simulink model "WaveletTraj"  (Simulink 10.1)
settings: Solver=FixedStepDiscrete  StartTime=0.0  StopTime=inf  FixedStep=Ts  RelTol=1e-3
PreLoadFcn:
  | load param
undefined symbols (not defined in the file or in its folder): c_maxsz, DiscIntNeverNeededParam, Dphival_fi, f, interp_gain, interp_uplim, phival_fi, Ts, tval_fi, w
libraries: simulink x36, dspsigops x24, dspindex x16, dspswit3 x12, simulink_extras x8
(part 4 of 4)

== system WaveletTraj/Wavelet Trajectory/TrajGen4/Compute Outputs/Compute Integral ==
  x : Inport
  max : Inport  Port=2
  min : Inport  Port=3
  Enable : EnablePort
  Compare To Zero : simulink/Logic and Bit Operations/Compare To Zero  SystemSampleTime=-1  relop=<  LogicOutDataTypeMode=boolean  ZeroCross=off
  Compare To Zero1 : simulink/Logic and Bit Operations/Compare To Zero  SystemSampleTime=-1  relop=>  LogicOutDataTypeMode=boolean  ZeroCross=off
  Discrete-Time Integrator : DiscreteIntegrator  IntegratorMethod=Integration: Trapezoidal  ExternalReset=level  InitialConditionSource=external  SampleTime=Ts  OutDataTypeStr=fixdt(1,w,f)  RndMeth=Nearest  SaturateOnIntegerOverflow=on  ICPrevOutput=DiscIntNeverNeededParam  ICPrevScaledInput=DiscIntNeverNeededParam
  Logical Operator : Logic  Operator=OR  IconShape=distinctive  AllPortsSameDT=off  OutDataTypeStr=boolean
  Logical Operator1 : Logic  IconShape=distinctive  AllPortsSameDT=off  OutDataTypeStr=boolean
  Logical Operator2 : Logic  IconShape=distinctive  AllPortsSameDT=off  OutDataTypeStr=boolean
  Logical Operator3 : Logic  Operator=OR  IconShape=distinctive  AllPortsSameDT=off  OutDataTypeStr=boolean
  Relational Operator1 : RelationalOperator  Operator=<=  OutDataTypeStr=boolean  RndMeth=Nearest
  Relational Operator2 : RelationalOperator  Operator=<=  OutDataTypeStr=boolean  RndMeth=Nearest
  S-R Flip-Flop : simulink_extras/Flip Flops/S-R Flip-Flop  SystemSampleTime=-1  initial_condition=0
  Sample and Hold1 : dspsigops/Sample and Hold  SystemSampleTime=-1  trig=Either edge  initCond=0  latchinput=off
  Sample and Hold2 : dspsigops/Sample and Hold  SystemSampleTime=-1  trig=Either edge  initCond=0  latchinput=off
  Saturation Dynamic : simulink/Discontinuities/Saturation Dynamic  SystemSampleTime=-1  OutMin=[]  OutMax=[]  OutDataTypeStr=fixdt(1,w,f)  OutputDataTypeScalingMode=Specify via dialog  OutDataType=fixdt(1,w,f)  OutScaling=[]  RndMeth=Nearest  DoSatur=on
  Terminator : Terminator
  Unit Delay : UnitDelay  SampleTime=-1
  Ix : Outport
  wires:
  Sample and Hold2/1 -> Logical Operator2/1
  Sample and Hold1/1 -> Logical Operator1/1
  Logical Operator3/1 -> S-R Flip-Flop/2
  Logical Operator2/1 -> Logical Operator3/2
  Logical Operator1/1 -> Logical Operator3/1
  Compare To Zero1/1 -> Logical Operator2/2
  Compare To Zero/1 -> Logical Operator1/2
  Logical Operator/1 -> Sample and Hold2/Trigger, Sample and Hold1/Trigger, S-R Flip-Flop/1
  S-R Flip-Flop/2 -> Terminator/1
  S-R Flip-Flop/1 -> Discrete-Time Integrator/2
  Unit Delay/1 -> Relational Operator2/1, Relational Operator1/2, Discrete-Time Integrator/3
  x/1 -> Compare To Zero1/1, Compare To Zero/1, Discrete-Time Integrator/1
  Saturation Dynamic/1 -> Unit Delay/1, Ix/1
  Discrete-Time Integrator/1 -> Saturation Dynamic/2
  Relational Operator2/1 -> Logical Operator/2, Sample and Hold2/1
  Relational Operator1/1 -> Sample and Hold1/1, Logical Operator/1
  min/1 -> Saturation Dynamic/3, Relational Operator2/2
  max/1 -> Saturation Dynamic/1, Relational Operator1/1

== system WaveletTraj/Wavelet Trajectory/TrajGen4/Compute Outputs/Rate Limiter1 ==
  up : Inport
  u : Inport  Port=2
  lo : Inport  Port=3
  Gain : Gain  Gain=1/Ts  ParamDataTypeStr=fixdt(1,w,f)  RndMeth=Nearest  SaturateOnIntegerOverflow=on  OutDataTypeStr=Inherit: Same as input
  Gain1 : Gain  Gain=Ts  ParamDataTypeStr=fixdt(1,w,f)  OutDataTypeStr=fixdt(1,w,f)  RndMeth=Nearest  SaturateOnIntegerOverflow=on
  Gain2 : Gain  Gain=Ts  ParamDataTypeStr=fixdt(1,w,f)  OutDataTypeStr=fixdt(1,w,f)  RndMeth=Nearest  SaturateOnIntegerOverflow=on
  Relational Operator : RelationalOperator  Operator=<  OutDataTypeStr=boolean  RndMeth=Nearest
  Relational Operator1 : RelationalOperator  Operator=>  OutDataTypeStr=boolean  RndMeth=Nearest
  Sum1 : Sum  Inputs=|++  OutDataTypeStr=fixdt(1,w,f)  RndMeth=Nearest  SaturateOnIntegerOverflow=on
  Sum2 : Sum  Inputs=|+-  OutDataTypeStr=fixdt(1,w,f)  RndMeth=Nearest  SaturateOnIntegerOverflow=on
  Sum3 : Sum  Inputs=|++  OutDataTypeStr=fixdt(1,w,f)  RndMeth=Nearest  SaturateOnIntegerOverflow=on
  Switch1 : Switch  Threshold=0.5  OutDataTypeStr=fixdt(1,w,f)  RndMeth=Nearest  SaturateOnIntegerOverflow=on
  Switch2 : Switch  Threshold=0.5  OutDataTypeStr=fixdt(1,w,f)  RndMeth=Nearest  SaturateOnIntegerOverflow=on
  Unit Delay : UnitDelay  SampleTime=-1
  y : Outport
  wires:
  Sum3/1 -> Switch2/3
  Gain2/1 -> Sum3/1
  lo/1 -> Gain2/1, Relational Operator1/2
  Relational Operator1/1 -> Switch2/2
  Switch2/1 -> Unit Delay/1, y/1
  Switch1/1 -> Switch2/1
  Sum1/1 -> Switch1/1
  Gain1/1 -> Sum1/1
  Relational Operator/1 -> Switch1/2
  up/1 -> Gain1/1, Relational Operator/1
  Gain/1 -> Relational Operator1/1, Relational Operator/2
  Unit Delay/1 -> Sum3/2, Sum1/2, Sum2/2
  Sum2/1 -> Gain/1
  u/1 -> Switch1/3, Sum2/1

== system WaveletTraj/Wavelet Trajectory/TrajGen4/Compute Outputs/Rate Limiter2 ==
  up : Inport
  u : Inport  Port=2
  lo : Inport  Port=3
  Gain : Gain  Gain=1/Ts  ParamDataTypeStr=fixdt(1,w,f)  RndMeth=Nearest  SaturateOnIntegerOverflow=on  OutDataTypeStr=Inherit: Same as input
  Gain1 : Gain  Gain=Ts  ParamDataTypeStr=fixdt(1,w,f)  OutDataTypeStr=fixdt(1,w,f)  RndMeth=Nearest  SaturateOnIntegerOverflow=on
  Gain2 : Gain  Gain=Ts  ParamDataTypeStr=fixdt(1,w,f)  OutDataTypeStr=fixdt(1,w,f)  RndMeth=Nearest  SaturateOnIntegerOverflow=on
  Relational Operator : RelationalOperator  Operator=<  OutDataTypeStr=boolean  RndMeth=Nearest
  Relational Operator1 : RelationalOperator  Operator=>  OutDataTypeStr=boolean  RndMeth=Nearest
  Sum1 : Sum  Inputs=|++  OutDataTypeStr=fixdt(1,w,f)  RndMeth=Nearest  SaturateOnIntegerOverflow=on
  Sum2 : Sum  Inputs=|+-  OutDataTypeStr=fixdt(1,w,f)  RndMeth=Nearest  SaturateOnIntegerOverflow=on
  Sum3 : Sum  Inputs=|++  OutDataTypeStr=fixdt(1,w,f)  RndMeth=Nearest  SaturateOnIntegerOverflow=on
  Switch1 : Switch  Threshold=0.5  OutDataTypeStr=fixdt(1,w,f)  RndMeth=Nearest  SaturateOnIntegerOverflow=on
  Switch2 : Switch  Threshold=0.5  OutDataTypeStr=fixdt(1,w,f)  RndMeth=Nearest  SaturateOnIntegerOverflow=on
  Unit Delay : UnitDelay  SampleTime=-1
  y : Outport
  wires:
  u/1 -> Sum2/1, Switch1/3
  Sum2/1 -> Gain/1
  Unit Delay/1 -> Sum2/2, Sum1/2, Sum3/2
  Gain/1 -> Relational Operator/2, Relational Operator1/1
  up/1 -> Relational Operator/1, Gain1/1
  Relational Operator/1 -> Switch1/2
  Gain1/1 -> Sum1/1
  Sum1/1 -> Switch1/1
  Switch1/1 -> Switch2/1
  Switch2/1 -> y/1, Unit Delay/1
  Relational Operator1/1 -> Switch2/2
  lo/1 -> Relational Operator1/2, Gain2/1
  Gain2/1 -> Sum3/1
  Sum3/1 -> Switch2/3

== system WaveletTraj/Wavelet Trajectory/TrajGen4/Compute Position/Position ==
  Res : Inport
  tau : Inport  Port=2
  c : Inport  Port=3
  N : Inport  Port=4
  Position : Subsystem  RTWFcnName=Trajectory_Position
  out : Outport
  wires:
  Res/1 -> Position/1(Res)
  tau/1 -> Position/2(tau)
  Position/1(out) -> out/1
  c/1 -> Position/3(c)
  N/1 -> Position/4(N)

== system WaveletTraj/Wavelet Trajectory/TrajGen4/Input Latching/Sample and Hold ==
  mode : Inport
  In : Inport  Port=2
  Trigger : TriggerPort  VariantControl=(inherit)  ZeroCross=off
  Constant : Constant  Value=2^3  OutDataTypeStr=fixdt(0,w,f)
  Constant1 : Constant  Value=2^4  OutDataTypeStr=fixdt(0,w,f)
  Data Type Conversion : DataTypeConversion  OutDataTypeStr=uint16  RndMeth=Ceiling  SaturateOnIntegerOverflow=on
  Multiport Switch : MultiPortSwitch  DataPortOrder=Zero-based contiguous  zeroidx=on  OutDataTypeStr=fixdt(0,w,f)  RndMeth=Nearest  SaturateOnIntegerOverflow=on
  " " : Outport  InitialOutput=initCond
  " 1" : Outport  Port=2  InitialOutput=initCond
  wires:
  Constant1/1 -> Multiport Switch/4
  Constant/1 -> Multiport Switch/3
  In/1 -> Multiport Switch/2
  mode/1 -> Multiport Switch/1
  Multiport Switch/1 -> Data Type Conversion/1, " "/1
  Data Type Conversion/1 -> " 1"/1

== system WaveletTraj/Wavelet Trajectory/TrajGen4/Input Latching/Sample and Hold2 ==
  In : Inport
  Trigger : TriggerPort  VariantControl=(inherit)  ZeroCross=off
  Data Type Conversion : DataTypeConversion  OutDataTypeStr=uint32  SaturateOnIntegerOverflow=on
  Gain : Gain  Gain=1/Ts  ParamDataTypeStr=fixdt(1,w,f)  OutDataTypeStr=fixdt(1,w,f)  RndMeth=Nearest  SaturateOnIntegerOverflow=on
  " " : Outport  InitialOutput=initCond
  wires:
  In/1 -> Gain/1
  Gain/1 -> Data Type Conversion/1
  Data Type Conversion/1 -> " "/1

== system WaveletTraj/Wavelet Trajectory/TrajGen4/Input Latching/Sample and Hold4 ==
  mode : Inport
  In : Inport  Port=2
  Trigger : TriggerPort  VariantControl=(inherit)  ZeroCross=off
  Multiport Switch : MultiPortSwitch  DataPortOrder=Zero-based contiguous  zeroidx=on  OutDataTypeStr=fixdt(1,w,f)  RndMeth=Nearest  SaturateOnIntegerOverflow=on
  constant : Constant  Value="[0.0156906989743308,  0.104549075132343,  0.277142440037961,  0.502199121925297,  0.726584938978675,  0.897421193763573,  0.982811374526835,  0.999579465917557,  1.00001660256494,  zeros(1,c_maxsz-9)]"  OutDataTypeStr=fixdt(1,w,f)
  constant1 : Constant  Value="[0.704980465851185,  0.994792363880808,  1.00001660256494*ones(1,15),  zeros(1,c_maxsz-17)]"  OutDataTypeStr=fixdt(1,w,f)
  " " : Outport  InitialOutput=initCond
  wires:
  constant1/1 -> Multiport Switch/4
  constant/1 -> Multiport Switch/3
  In/1 -> Multiport Switch/2
  mode/1 -> Multiport Switch/1
  Multiport Switch/1 -> " "/1

== system WaveletTraj/Wavelet Trajectory/TrajGen4/Input Latching/Sample and Hold5 ==
  mode : Inport
  x0 : Inport  Port=2
  xf : Inport  Port=3
  Trigger : TriggerPort  VariantControl=(inherit)  ZeroCross=off
  Constant : Constant  OutDataTypeStr=fixdt(1,w,f)
  Sum2 : Sum  Inputs=-+|  OutDataTypeStr=fixdt(1,w,f)  RndMeth=Nearest  SaturateOnIntegerOverflow=on
  Switch1 : Switch  Threshold=0.5  OutDataTypeStr=fixdt(1,w,f)  RndMeth=Nearest  SaturateOnIntegerOverflow=on
  " " : Outport  InitialOutput=initCond
  wires:
  Constant/1 -> Switch1/3
  Switch1/1 -> " "/1
  Sum2/1 -> Switch1/1
  mode/1 -> Switch1/2
  xf/1 -> Sum2/2
  x0/1 -> Sum2/1

== system WaveletTraj/Wavelet Trajectory/TrajGen1/Compute Join Coeffs/Derivative1 in tau/Derivative ==
  Res : Inport  PortDimensions=1
  tau : Inport  Port=2  PortDimensions=1
  c : Inport  Port=3  PortDimensions=c_maxsz
  N : Inport  Port=4  PortDimensions=1
  For Iterator : ForIterator  ResetStates=reset  IterationSource=external  IndexMode=Zero-based  IterationVariableDataType=int8
  Lookup Table : Lookup  InputValues=tval_fi  Table=Dphival_fi  LookUpMeth=Interpolation-Use End Values  RndMeth=Nearest  SaturateOnIntegerOverflow=on
  Memory : Memory  InheritSampleTime=on
  Product : Product  OutDataTypeStr=fixdt(1,w,f)  RndMeth=Nearest  SaturateOnIntegerOverflow=on
  Product2 : Product  Inputs=3  OutDataTypeStr=fixdt(1,w,f)  RndMeth=Nearest  SaturateOnIntegerOverflow=on
  Selector : Selector  IndexMode=Zero-based  InputPortWidth=c_maxsz  IndexOptions=Index vector (port)  Indices=[1 3]  OutputSizes=1
  Sum : Sum  Inputs=|+-  OutDataTypeStr=fixdt(1,w,f)  RndMeth=Nearest  SaturateOnIntegerOverflow=on
  Sum1 : Sum  Inputs=|++  OutDataTypeStr=fixdt(1,w,f)  RndMeth=Nearest  SaturateOnIntegerOverflow=on
  Dout : Outport  PortDimensions=1  InitialOutput=0
  wires:
  Product2/1 -> Sum1/1
  Selector/1 -> Product2/3
  Lookup Table/1 -> Product2/2
  Sum1/1 -> Memory/1, Dout/1
  Memory/1 -> Sum1/2
  c/1 -> Selector/1
  For Iterator/1 -> Selector/2, Sum/2
  N/1 -> For Iterator/1
  Product/1 -> Sum/1
  Sum/1 -> Lookup Table/1
  Res/1 -> Product2/1, Product/1
  tau/1 -> Product/2

== system WaveletTraj/Wavelet Trajectory/TrajGen1/Compute Join Coeffs/Derivative2 in 0/Derivative ==
  Res : Inport  PortDimensions=1
  tau : Inport  Port=2  PortDimensions=1
  c : Inport  Port=3  PortDimensions=c_maxsz
  N : Inport  Port=4  PortDimensions=1
  For Iterator : ForIterator  ResetStates=reset  IterationSource=external  IndexMode=Zero-based  IterationVariableDataType=int8
  Lookup Table : Lookup  InputValues=tval_fi  Table=Dphival_fi  LookUpMeth=Interpolation-Use End Values  RndMeth=Nearest  SaturateOnIntegerOverflow=on
  Memory : Memory  InheritSampleTime=on
  Product : Product  OutDataTypeStr=fixdt(1,w,f)  RndMeth=Nearest  SaturateOnIntegerOverflow=on
  Product2 : Product  Inputs=3  OutDataTypeStr=fixdt(1,w,f)  RndMeth=Nearest  SaturateOnIntegerOverflow=on
  Selector : Selector  IndexMode=Zero-based  InputPortWidth=c_maxsz  IndexOptions=Index vector (port)  Indices=[1 3]  OutputSizes=1
  Sum : Sum  Inputs=|+-  OutDataTypeStr=fixdt(1,w,f)  RndMeth=Nearest  SaturateOnIntegerOverflow=on
  Sum1 : Sum  Inputs=|++  OutDataTypeStr=fixdt(1,w,f)  RndMeth=Nearest  SaturateOnIntegerOverflow=on
  Dout : Outport  PortDimensions=1  InitialOutput=0
  wires:
  tau/1 -> Product/2
  Res/1 -> Product/1, Product2/1
  Sum/1 -> Lookup Table/1
  Product/1 -> Sum/1
  N/1 -> For Iterator/1
  For Iterator/1 -> Sum/2, Selector/2
  c/1 -> Selector/1
  Memory/1 -> Sum1/2
  Sum1/1 -> Dout/1, Memory/1
  Lookup Table/1 -> Product2/2
  Selector/1 -> Product2/3
  Product2/1 -> Sum1/1

== system WaveletTraj/Wavelet Trajectory/TrajGen1/Compute Join Coeffs/Derivative2 in tau1/Derivative ==
  Res : Inport  PortDimensions=1
  tau : Inport  Port=2  PortDimensions=1
  c : Inport  Port=3  PortDimensions=c_maxsz
  N : Inport  Port=4  PortDimensions=1
  For Iterator : ForIterator  ResetStates=reset  IterationSource=external  IndexMode=Zero-based  IterationVariableDataType=int8
  Lookup Table : Lookup  InputValues=tval_fi  Table=Dphival_fi  LookUpMeth=Interpolation-Use End Values  RndMeth=Nearest  SaturateOnIntegerOverflow=on
  Memory : Memory  InheritSampleTime=on
  Product : Product  OutDataTypeStr=fixdt(1,w,f)  RndMeth=Nearest  SaturateOnIntegerOverflow=on
  Product2 : Product  Inputs=3  OutDataTypeStr=fixdt(1,w,f)  RndMeth=Nearest  SaturateOnIntegerOverflow=on
  Selector : Selector  IndexMode=Zero-based  InputPortWidth=c_maxsz  IndexOptions=Index vector (port)  Indices=[1 3]  OutputSizes=1
  Sum : Sum  Inputs=|+-  OutDataTypeStr=fixdt(1,w,f)  RndMeth=Nearest  SaturateOnIntegerOverflow=on
  Sum1 : Sum  Inputs=|++  OutDataTypeStr=fixdt(1,w,f)  RndMeth=Nearest  SaturateOnIntegerOverflow=on
  Dout : Outport  PortDimensions=1  InitialOutput=0
  wires:
  Product2/1 -> Sum1/1
  Selector/1 -> Product2/3
  Lookup Table/1 -> Product2/2
  Sum1/1 -> Memory/1, Dout/1
  Memory/1 -> Sum1/2
  c/1 -> Selector/1
  For Iterator/1 -> Selector/2, Sum/2
  N/1 -> For Iterator/1
  Product/1 -> Sum/1
  Sum/1 -> Lookup Table/1
  Res/1 -> Product2/1, Product/1
  tau/1 -> Product/2

== system WaveletTraj/Wavelet Trajectory/TrajGen1/Compute Join Coeffs/Position2 in tau1/Position ==
  Res : Inport  PortDimensions=1
  tau : Inport  Port=2  PortDimensions=1
  c : Inport  Port=3  PortDimensions=c_maxsz
  N : Inport  Port=4  PortDimensions=1
  For Iterator : ForIterator  ResetStates=reset  IterationSource=external  IndexMode=Zero-based  IterationVariableDataType=int8
  Lookup Table : Lookup  InputValues=tval_fi  Table=phival_fi  LookUpMeth=Interpolation-Use End Values  RndMeth=Nearest  SaturateOnIntegerOverflow=on
  Memory : Memory  InheritSampleTime=on
  Product : Product  OutDataTypeStr=fixdt(1,w,f)  RndMeth=Nearest  SaturateOnIntegerOverflow=on
  Product1 : Product  OutDataTypeStr=fixdt(1,w,f)  RndMeth=Nearest  SaturateOnIntegerOverflow=on
  Selector : Selector  IndexMode=Zero-based  InputPortWidth=c_maxsz  IndexOptions=Index vector (port)  Indices=[1 3]  OutputSizes=1
  Sum : Sum  Inputs=|+-  OutDataTypeStr=fixdt(1,w,f)  RndMeth=Nearest  SaturateOnIntegerOverflow=on
  Sum1 : Sum  Inputs=|++  OutDataTypeStr=fixdt(1,w,f)  RndMeth=Nearest  SaturateOnIntegerOverflow=on
  out : Outport  PortDimensions=1  InitialOutput=0
  wires:
  tau/1 -> Product/2
  Res/1 -> Product/1
  Sum/1 -> Lookup Table/1
  Product/1 -> Sum/1
  N/1 -> For Iterator/1
  For Iterator/1 -> Sum/2, Selector/2
  Lookup Table/1 -> Product1/1
  c/1 -> Selector/1
  Selector/1 -> Product1/2
  Product1/1 -> Sum1/1
  Memory/1 -> Sum1/2
  Sum1/1 -> out/1, Memory/1

== system WaveletTraj/Wavelet Trajectory/TrajGen1/Compute Position/Position/Position ==
  Res : Inport  PortDimensions=1
  tau : Inport  Port=2  PortDimensions=1
  c : Inport  Port=3  PortDimensions=c_maxsz
  N : Inport  Port=4  PortDimensions=1
  For Iterator : ForIterator  ResetStates=reset  IterationSource=external  IndexMode=Zero-based  IterationVariableDataType=int8
  Lookup Table : Lookup  InputValues=tval_fi  Table=phival_fi  LookUpMeth=Interpolation-Use End Values  RndMeth=Nearest  SaturateOnIntegerOverflow=on
  Memory : Memory  InheritSampleTime=on
  Product : Product  OutDataTypeStr=fixdt(1,w,f)  RndMeth=Nearest  SaturateOnIntegerOverflow=on
  Product1 : Product  OutDataTypeStr=fixdt(1,w,f)  RndMeth=Nearest  SaturateOnIntegerOverflow=on
  Selector : Selector  IndexMode=Zero-based  InputPortWidth=c_maxsz  IndexOptions=Index vector (port)  Indices=[1 3]  OutputSizes=1
  Sum : Sum  Inputs=|+-  OutDataTypeStr=fixdt(1,w,f)  RndMeth=Nearest  SaturateOnIntegerOverflow=on
  Sum1 : Sum  Inputs=|++  OutDataTypeStr=fixdt(1,w,f)  RndMeth=Nearest  SaturateOnIntegerOverflow=on
  out : Outport  PortDimensions=1  InitialOutput=0
  wires:
  Sum1/1 -> Memory/1, out/1
  Memory/1 -> Sum1/2
  Product1/1 -> Sum1/1
  Selector/1 -> Product1/2
  c/1 -> Selector/1
  Lookup Table/1 -> Product1/1
  For Iterator/1 -> Selector/2, Sum/2
  N/1 -> For Iterator/1
  Product/1 -> Sum/1
  Sum/1 -> Lookup Table/1
  Res/1 -> Product/1
  tau/1 -> Product/2

== system WaveletTraj/Wavelet Trajectory/TrajGen2/Compute Join Coeffs/Derivative1 in tau/Derivative ==
  Res : Inport  PortDimensions=1
  tau : Inport  Port=2  PortDimensions=1
  c : Inport  Port=3  PortDimensions=c_maxsz
  N : Inport  Port=4  PortDimensions=1
  For Iterator : ForIterator  ResetStates=reset  IterationSource=external  IndexMode=Zero-based  IterationVariableDataType=int8
  Lookup Table : Lookup  InputValues=tval_fi  Table=Dphival_fi  LookUpMeth=Interpolation-Use End Values  RndMeth=Nearest  SaturateOnIntegerOverflow=on
  Memory : Memory  InheritSampleTime=on
  Product : Product  OutDataTypeStr=fixdt(1,w,f)  RndMeth=Nearest  SaturateOnIntegerOverflow=on
  Product2 : Product  Inputs=3  OutDataTypeStr=fixdt(1,w,f)  RndMeth=Nearest  SaturateOnIntegerOverflow=on
  Selector : Selector  IndexMode=Zero-based  InputPortWidth=c_maxsz  IndexOptions=Index vector (port)  Indices=[1 3]  OutputSizes=1
  Sum : Sum  Inputs=|+-  OutDataTypeStr=fixdt(1,w,f)  RndMeth=Nearest  SaturateOnIntegerOverflow=on
  Sum1 : Sum  Inputs=|++  OutDataTypeStr=fixdt(1,w,f)  RndMeth=Nearest  SaturateOnIntegerOverflow=on
  Dout : Outport  PortDimensions=1  InitialOutput=0
  wires:
  tau/1 -> Product/2
  Res/1 -> Product/1, Product2/1
  Sum/1 -> Lookup Table/1
  Product/1 -> Sum/1
  N/1 -> For Iterator/1
  For Iterator/1 -> Sum/2, Selector/2
  c/1 -> Selector/1
  Memory/1 -> Sum1/2
  Sum1/1 -> Dout/1, Memory/1
  Lookup Table/1 -> Product2/2
  Selector/1 -> Product2/3
  Product2/1 -> Sum1/1

== system WaveletTraj/Wavelet Trajectory/TrajGen2/Compute Join Coeffs/Derivative2 in 0/Derivative ==
  Res : Inport  PortDimensions=1
  tau : Inport  Port=2  PortDimensions=1
  c : Inport  Port=3  PortDimensions=c_maxsz
  N : Inport  Port=4  PortDimensions=1
  For Iterator : ForIterator  ResetStates=reset  IterationSource=external  IndexMode=Zero-based  IterationVariableDataType=int8
  Lookup Table : Lookup  InputValues=tval_fi  Table=Dphival_fi  LookUpMeth=Interpolation-Use End Values  RndMeth=Nearest  SaturateOnIntegerOverflow=on
  Memory : Memory  InheritSampleTime=on
  Product : Product  OutDataTypeStr=fixdt(1,w,f)  RndMeth=Nearest  SaturateOnIntegerOverflow=on
  Product2 : Product  Inputs=3  OutDataTypeStr=fixdt(1,w,f)  RndMeth=Nearest  SaturateOnIntegerOverflow=on
  Selector : Selector  IndexMode=Zero-based  InputPortWidth=c_maxsz  IndexOptions=Index vector (port)  Indices=[1 3]  OutputSizes=1
  Sum : Sum  Inputs=|+-  OutDataTypeStr=fixdt(1,w,f)  RndMeth=Nearest  SaturateOnIntegerOverflow=on
  Sum1 : Sum  Inputs=|++  OutDataTypeStr=fixdt(1,w,f)  RndMeth=Nearest  SaturateOnIntegerOverflow=on
  Dout : Outport  PortDimensions=1  InitialOutput=0
  wires:
  Product2/1 -> Sum1/1
  Selector/1 -> Product2/3
  Lookup Table/1 -> Product2/2
  Sum1/1 -> Memory/1, Dout/1
  Memory/1 -> Sum1/2
  c/1 -> Selector/1
  For Iterator/1 -> Selector/2, Sum/2
  N/1 -> For Iterator/1
  Product/1 -> Sum/1
  Sum/1 -> Lookup Table/1
  Res/1 -> Product2/1, Product/1
  tau/1 -> Product/2

== system WaveletTraj/Wavelet Trajectory/TrajGen2/Compute Join Coeffs/Derivative2 in tau1/Derivative ==
  Res : Inport  PortDimensions=1
  tau : Inport  Port=2  PortDimensions=1
  c : Inport  Port=3  PortDimensions=c_maxsz
  N : Inport  Port=4  PortDimensions=1
  For Iterator : ForIterator  ResetStates=reset  IterationSource=external  IndexMode=Zero-based  IterationVariableDataType=int8
  Lookup Table : Lookup  InputValues=tval_fi  Table=Dphival_fi  LookUpMeth=Interpolation-Use End Values  RndMeth=Nearest  SaturateOnIntegerOverflow=on
  Memory : Memory  InheritSampleTime=on
  Product : Product  OutDataTypeStr=fixdt(1,w,f)  RndMeth=Nearest  SaturateOnIntegerOverflow=on
  Product2 : Product  Inputs=3  OutDataTypeStr=fixdt(1,w,f)  RndMeth=Nearest  SaturateOnIntegerOverflow=on
  Selector : Selector  IndexMode=Zero-based  InputPortWidth=c_maxsz  IndexOptions=Index vector (port)  Indices=[1 3]  OutputSizes=1
  Sum : Sum  Inputs=|+-  OutDataTypeStr=fixdt(1,w,f)  RndMeth=Nearest  SaturateOnIntegerOverflow=on
  Sum1 : Sum  Inputs=|++  OutDataTypeStr=fixdt(1,w,f)  RndMeth=Nearest  SaturateOnIntegerOverflow=on
  Dout : Outport  PortDimensions=1  InitialOutput=0
  wires:
  tau/1 -> Product/2
  Res/1 -> Product/1, Product2/1
  Sum/1 -> Lookup Table/1
  Product/1 -> Sum/1
  N/1 -> For Iterator/1
  For Iterator/1 -> Sum/2, Selector/2
  c/1 -> Selector/1
  Memory/1 -> Sum1/2
  Sum1/1 -> Dout/1, Memory/1
  Lookup Table/1 -> Product2/2
  Selector/1 -> Product2/3
  Product2/1 -> Sum1/1

== system WaveletTraj/Wavelet Trajectory/TrajGen2/Compute Join Coeffs/Position2 in tau1/Position ==
  Res : Inport  PortDimensions=1
  tau : Inport  Port=2  PortDimensions=1
  c : Inport  Port=3  PortDimensions=c_maxsz
  N : Inport  Port=4  PortDimensions=1
  For Iterator : ForIterator  ResetStates=reset  IterationSource=external  IndexMode=Zero-based  IterationVariableDataType=int8
  Lookup Table : Lookup  InputValues=tval_fi  Table=phival_fi  LookUpMeth=Interpolation-Use End Values  RndMeth=Nearest  SaturateOnIntegerOverflow=on
  Memory : Memory  InheritSampleTime=on
  Product : Product  OutDataTypeStr=fixdt(1,w,f)  RndMeth=Nearest  SaturateOnIntegerOverflow=on
  Product1 : Product  OutDataTypeStr=fixdt(1,w,f)  RndMeth=Nearest  SaturateOnIntegerOverflow=on
  Selector : Selector  IndexMode=Zero-based  InputPortWidth=c_maxsz  IndexOptions=Index vector (port)  Indices=[1 3]  OutputSizes=1
  Sum : Sum  Inputs=|+-  OutDataTypeStr=fixdt(1,w,f)  RndMeth=Nearest  SaturateOnIntegerOverflow=on
  Sum1 : Sum  Inputs=|++  OutDataTypeStr=fixdt(1,w,f)  RndMeth=Nearest  SaturateOnIntegerOverflow=on
  out : Outport  PortDimensions=1  InitialOutput=0
  wires:
  Sum1/1 -> Memory/1, out/1
  Memory/1 -> Sum1/2
  Product1/1 -> Sum1/1
  Selector/1 -> Product1/2
  c/1 -> Selector/1
  Lookup Table/1 -> Product1/1
  For Iterator/1 -> Selector/2, Sum/2
  N/1 -> For Iterator/1
  Product/1 -> Sum/1
  Sum/1 -> Lookup Table/1
  Res/1 -> Product/1
  tau/1 -> Product/2

== system WaveletTraj/Wavelet Trajectory/TrajGen2/Compute Position/Position/Position ==
  Res : Inport  PortDimensions=1
  tau : Inport  Port=2  PortDimensions=1
  c : Inport  Port=3  PortDimensions=c_maxsz
  N : Inport  Port=4  PortDimensions=1
  For Iterator : ForIterator  ResetStates=reset  IterationSource=external  IndexMode=Zero-based  IterationVariableDataType=int8
  Lookup Table : Lookup  InputValues=tval_fi  Table=phival_fi  LookUpMeth=Interpolation-Use End Values  RndMeth=Nearest  SaturateOnIntegerOverflow=on
  Memory : Memory  InheritSampleTime=on
  Product : Product  OutDataTypeStr=fixdt(1,w,f)  RndMeth=Nearest  SaturateOnIntegerOverflow=on
  Product1 : Product  OutDataTypeStr=fixdt(1,w,f)  RndMeth=Nearest  SaturateOnIntegerOverflow=on
  Selector : Selector  IndexMode=Zero-based  InputPortWidth=c_maxsz  IndexOptions=Index vector (port)  Indices=[1 3]  OutputSizes=1
  Sum : Sum  Inputs=|+-  OutDataTypeStr=fixdt(1,w,f)  RndMeth=Nearest  SaturateOnIntegerOverflow=on
  Sum1 : Sum  Inputs=|++  OutDataTypeStr=fixdt(1,w,f)  RndMeth=Nearest  SaturateOnIntegerOverflow=on
  out : Outport  PortDimensions=1  InitialOutput=0
  wires:
  tau/1 -> Product/2
  Res/1 -> Product/1
  Sum/1 -> Lookup Table/1
  Product/1 -> Sum/1
  N/1 -> For Iterator/1
  For Iterator/1 -> Sum/2, Selector/2
  Lookup Table/1 -> Product1/1
  c/1 -> Selector/1
  Selector/1 -> Product1/2
  Product1/1 -> Sum1/1
  Memory/1 -> Sum1/2
  Sum1/1 -> out/1, Memory/1

== system WaveletTraj/Wavelet Trajectory/TrajGen3/Compute Join Coeffs/Derivative1 in tau/Derivative ==
  Res : Inport  PortDimensions=1
  tau : Inport  Port=2  PortDimensions=1
  c : Inport  Port=3  PortDimensions=c_maxsz
  N : Inport  Port=4  PortDimensions=1
  For Iterator : ForIterator  ResetStates=reset  IterationSource=external  IndexMode=Zero-based  IterationVariableDataType=int8
  Lookup Table : Lookup  InputValues=tval_fi  Table=Dphival_fi  LookUpMeth=Interpolation-Use End Values  RndMeth=Nearest  SaturateOnIntegerOverflow=on
  Memory : Memory  InheritSampleTime=on
  Product : Product  OutDataTypeStr=fixdt(1,w,f)  RndMeth=Nearest  SaturateOnIntegerOverflow=on
  Product2 : Product  Inputs=3  OutDataTypeStr=fixdt(1,w,f)  RndMeth=Nearest  SaturateOnIntegerOverflow=on
  Selector : Selector  IndexMode=Zero-based  InputPortWidth=c_maxsz  IndexOptions=Index vector (port)  Indices=[1 3]  OutputSizes=1
  Sum : Sum  Inputs=|+-  OutDataTypeStr=fixdt(1,w,f)  RndMeth=Nearest  SaturateOnIntegerOverflow=on
  Sum1 : Sum  Inputs=|++  OutDataTypeStr=fixdt(1,w,f)  RndMeth=Nearest  SaturateOnIntegerOverflow=on
  Dout : Outport  PortDimensions=1  InitialOutput=0
  wires:
  Product2/1 -> Sum1/1
  Selector/1 -> Product2/3
  Lookup Table/1 -> Product2/2
  Sum1/1 -> Memory/1, Dout/1
  Memory/1 -> Sum1/2
  c/1 -> Selector/1
  For Iterator/1 -> Selector/2, Sum/2
  N/1 -> For Iterator/1
  Product/1 -> Sum/1
  Sum/1 -> Lookup Table/1
  Res/1 -> Product2/1, Product/1
  tau/1 -> Product/2

== system WaveletTraj/Wavelet Trajectory/TrajGen3/Compute Join Coeffs/Derivative2 in 0/Derivative ==
  Res : Inport  PortDimensions=1
  tau : Inport  Port=2  PortDimensions=1
  c : Inport  Port=3  PortDimensions=c_maxsz
  N : Inport  Port=4  PortDimensions=1
  For Iterator : ForIterator  ResetStates=reset  IterationSource=external  IndexMode=Zero-based  IterationVariableDataType=int8
  Lookup Table : Lookup  InputValues=tval_fi  Table=Dphival_fi  LookUpMeth=Interpolation-Use End Values  RndMeth=Nearest  SaturateOnIntegerOverflow=on
  Memory : Memory  InheritSampleTime=on
  Product : Product  OutDataTypeStr=fixdt(1,w,f)  RndMeth=Nearest  SaturateOnIntegerOverflow=on
  Product2 : Product  Inputs=3  OutDataTypeStr=fixdt(1,w,f)  RndMeth=Nearest  SaturateOnIntegerOverflow=on
  Selector : Selector  IndexMode=Zero-based  InputPortWidth=c_maxsz  IndexOptions=Index vector (port)  Indices=[1 3]  OutputSizes=1
  Sum : Sum  Inputs=|+-  OutDataTypeStr=fixdt(1,w,f)  RndMeth=Nearest  SaturateOnIntegerOverflow=on
  Sum1 : Sum  Inputs=|++  OutDataTypeStr=fixdt(1,w,f)  RndMeth=Nearest  SaturateOnIntegerOverflow=on
  Dout : Outport  PortDimensions=1  InitialOutput=0
  wires:
  tau/1 -> Product/2
  Res/1 -> Product/1, Product2/1
  Sum/1 -> Lookup Table/1
  Product/1 -> Sum/1
  N/1 -> For Iterator/1
  For Iterator/1 -> Sum/2, Selector/2
  c/1 -> Selector/1
  Memory/1 -> Sum1/2
  Sum1/1 -> Dout/1, Memory/1
  Lookup Table/1 -> Product2/2
  Selector/1 -> Product2/3
  Product2/1 -> Sum1/1

== system WaveletTraj/Wavelet Trajectory/TrajGen3/Compute Join Coeffs/Derivative2 in tau1/Derivative ==
  Res : Inport  PortDimensions=1
  tau : Inport  Port=2  PortDimensions=1
  c : Inport  Port=3  PortDimensions=c_maxsz
  N : Inport  Port=4  PortDimensions=1
  For Iterator : ForIterator  ResetStates=reset  IterationSource=external  IndexMode=Zero-based  IterationVariableDataType=int8
  Lookup Table : Lookup  InputValues=tval_fi  Table=Dphival_fi  LookUpMeth=Interpolation-Use End Values  RndMeth=Nearest  SaturateOnIntegerOverflow=on
  Memory : Memory  InheritSampleTime=on
  Product : Product  OutDataTypeStr=fixdt(1,w,f)  RndMeth=Nearest  SaturateOnIntegerOverflow=on
  Product2 : Product  Inputs=3  OutDataTypeStr=fixdt(1,w,f)  RndMeth=Nearest  SaturateOnIntegerOverflow=on
  Selector : Selector  IndexMode=Zero-based  InputPortWidth=c_maxsz  IndexOptions=Index vector (port)  Indices=[1 3]  OutputSizes=1
  Sum : Sum  Inputs=|+-  OutDataTypeStr=fixdt(1,w,f)  RndMeth=Nearest  SaturateOnIntegerOverflow=on
  Sum1 : Sum  Inputs=|++  OutDataTypeStr=fixdt(1,w,f)  RndMeth=Nearest  SaturateOnIntegerOverflow=on
  Dout : Outport  PortDimensions=1  InitialOutput=0
  wires:
  Product2/1 -> Sum1/1
  Selector/1 -> Product2/3
  Lookup Table/1 -> Product2/2
  Sum1/1 -> Memory/1, Dout/1
  Memory/1 -> Sum1/2
  c/1 -> Selector/1
  For Iterator/1 -> Selector/2, Sum/2
  N/1 -> For Iterator/1
  Product/1 -> Sum/1
  Sum/1 -> Lookup Table/1
  Res/1 -> Product2/1, Product/1
  tau/1 -> Product/2

== system WaveletTraj/Wavelet Trajectory/TrajGen3/Compute Join Coeffs/Position2 in tau1/Position ==
  Res : Inport  PortDimensions=1
  tau : Inport  Port=2  PortDimensions=1
  c : Inport  Port=3  PortDimensions=c_maxsz
  N : Inport  Port=4  PortDimensions=1
  For Iterator : ForIterator  ResetStates=reset  IterationSource=external  IndexMode=Zero-based  IterationVariableDataType=int8
  Lookup Table : Lookup  InputValues=tval_fi  Table=phival_fi  LookUpMeth=Interpolation-Use End Values  RndMeth=Nearest  SaturateOnIntegerOverflow=on
  Memory : Memory  InheritSampleTime=on
  Product : Product  OutDataTypeStr=fixdt(1,w,f)  RndMeth=Nearest  SaturateOnIntegerOverflow=on
  Product1 : Product  OutDataTypeStr=fixdt(1,w,f)  RndMeth=Nearest  SaturateOnIntegerOverflow=on
  Selector : Selector  IndexMode=Zero-based  InputPortWidth=c_maxsz  IndexOptions=Index vector (port)  Indices=[1 3]  OutputSizes=1
  Sum : Sum  Inputs=|+-  OutDataTypeStr=fixdt(1,w,f)  RndMeth=Nearest  SaturateOnIntegerOverflow=on
  Sum1 : Sum  Inputs=|++  OutDataTypeStr=fixdt(1,w,f)  RndMeth=Nearest  SaturateOnIntegerOverflow=on
  out : Outport  PortDimensions=1  InitialOutput=0
  wires:
  tau/1 -> Product/2
  Res/1 -> Product/1
  Sum/1 -> Lookup Table/1
  Product/1 -> Sum/1
  N/1 -> For Iterator/1
  For Iterator/1 -> Sum/2, Selector/2
  Lookup Table/1 -> Product1/1
  c/1 -> Selector/1
  Selector/1 -> Product1/2
  Product1/1 -> Sum1/1
  Memory/1 -> Sum1/2
  Sum1/1 -> out/1, Memory/1

== system WaveletTraj/Wavelet Trajectory/TrajGen3/Compute Position/Position/Position ==
  Res : Inport  PortDimensions=1
  tau : Inport  Port=2  PortDimensions=1
  c : Inport  Port=3  PortDimensions=c_maxsz
  N : Inport  Port=4  PortDimensions=1
  For Iterator : ForIterator  ResetStates=reset  IterationSource=external  IndexMode=Zero-based  IterationVariableDataType=int8
  Lookup Table : Lookup  InputValues=tval_fi  Table=phival_fi  LookUpMeth=Interpolation-Use End Values  RndMeth=Nearest  SaturateOnIntegerOverflow=on
  Memory : Memory  InheritSampleTime=on
  Product : Product  OutDataTypeStr=fixdt(1,w,f)  RndMeth=Nearest  SaturateOnIntegerOverflow=on
  Product1 : Product  OutDataTypeStr=fixdt(1,w,f)  RndMeth=Nearest  SaturateOnIntegerOverflow=on
  Selector : Selector  IndexMode=Zero-based  InputPortWidth=c_maxsz  IndexOptions=Index vector (port)  Indices=[1 3]  OutputSizes=1
  Sum : Sum  Inputs=|+-  OutDataTypeStr=fixdt(1,w,f)  RndMeth=Nearest  SaturateOnIntegerOverflow=on
  Sum1 : Sum  Inputs=|++  OutDataTypeStr=fixdt(1,w,f)  RndMeth=Nearest  SaturateOnIntegerOverflow=on
  out : Outport  PortDimensions=1  InitialOutput=0
  wires:
  Sum1/1 -> Memory/1, out/1
  Memory/1 -> Sum1/2
  Product1/1 -> Sum1/1
  Selector/1 -> Product1/2
  c/1 -> Selector/1
  Lookup Table/1 -> Product1/1
  For Iterator/1 -> Selector/2, Sum/2
  N/1 -> For Iterator/1
  Product/1 -> Sum/1
  Sum/1 -> Lookup Table/1
  Res/1 -> Product/1
  tau/1 -> Product/2

== system WaveletTraj/Wavelet Trajectory/TrajGen4/Compute Join Coeffs/Derivative1 in tau/Derivative ==
  Res : Inport  PortDimensions=1
  tau : Inport  Port=2  PortDimensions=1
  c : Inport  Port=3  PortDimensions=c_maxsz
  N : Inport  Port=4  PortDimensions=1
  For Iterator : ForIterator  ResetStates=reset  IterationSource=external  IndexMode=Zero-based  IterationVariableDataType=int8
  Lookup Table : Lookup  InputValues=tval_fi  Table=Dphival_fi  LookUpMeth=Interpolation-Use End Values  RndMeth=Nearest  SaturateOnIntegerOverflow=on
  Memory : Memory  InheritSampleTime=on
  Product : Product  OutDataTypeStr=fixdt(1,w,f)  RndMeth=Nearest  SaturateOnIntegerOverflow=on
  Product2 : Product  Inputs=3  OutDataTypeStr=fixdt(1,w,f)  RndMeth=Nearest  SaturateOnIntegerOverflow=on
  Selector : Selector  IndexMode=Zero-based  InputPortWidth=c_maxsz  IndexOptions=Index vector (port)  Indices=[1 3]  OutputSizes=1
  Sum : Sum  Inputs=|+-  OutDataTypeStr=fixdt(1,w,f)  RndMeth=Nearest  SaturateOnIntegerOverflow=on
  Sum1 : Sum  Inputs=|++  OutDataTypeStr=fixdt(1,w,f)  RndMeth=Nearest  SaturateOnIntegerOverflow=on
  Dout : Outport  PortDimensions=1  InitialOutput=0
  wires:
  tau/1 -> Product/2
  Res/1 -> Product/1, Product2/1
  Sum/1 -> Lookup Table/1
  Product/1 -> Sum/1
  N/1 -> For Iterator/1
  For Iterator/1 -> Sum/2, Selector/2
  c/1 -> Selector/1
  Memory/1 -> Sum1/2
  Sum1/1 -> Dout/1, Memory/1
  Lookup Table/1 -> Product2/2
  Selector/1 -> Product2/3
  Product2/1 -> Sum1/1

== system WaveletTraj/Wavelet Trajectory/TrajGen4/Compute Join Coeffs/Derivative2 in 0/Derivative ==
  Res : Inport  PortDimensions=1
  tau : Inport  Port=2  PortDimensions=1
  c : Inport  Port=3  PortDimensions=c_maxsz
  N : Inport  Port=4  PortDimensions=1
  For Iterator : ForIterator  ResetStates=reset  IterationSource=external  IndexMode=Zero-based  IterationVariableDataType=int8
  Lookup Table : Lookup  InputValues=tval_fi  Table=Dphival_fi  LookUpMeth=Interpolation-Use End Values  RndMeth=Nearest  SaturateOnIntegerOverflow=on
  Memory : Memory  InheritSampleTime=on
  Product : Product  OutDataTypeStr=fixdt(1,w,f)  RndMeth=Nearest  SaturateOnIntegerOverflow=on
  Product2 : Product  Inputs=3  OutDataTypeStr=fixdt(1,w,f)  RndMeth=Nearest  SaturateOnIntegerOverflow=on
  Selector : Selector  IndexMode=Zero-based  InputPortWidth=c_maxsz  IndexOptions=Index vector (port)  Indices=[1 3]  OutputSizes=1
  Sum : Sum  Inputs=|+-  OutDataTypeStr=fixdt(1,w,f)  RndMeth=Nearest  SaturateOnIntegerOverflow=on
  Sum1 : Sum  Inputs=|++  OutDataTypeStr=fixdt(1,w,f)  RndMeth=Nearest  SaturateOnIntegerOverflow=on
  Dout : Outport  PortDimensions=1  InitialOutput=0
  wires:
  Product2/1 -> Sum1/1
  Selector/1 -> Product2/3
  Lookup Table/1 -> Product2/2
  Sum1/1 -> Memory/1, Dout/1
  Memory/1 -> Sum1/2
  c/1 -> Selector/1
  For Iterator/1 -> Selector/2, Sum/2
  N/1 -> For Iterator/1
  Product/1 -> Sum/1
  Sum/1 -> Lookup Table/1
  Res/1 -> Product2/1, Product/1
  tau/1 -> Product/2

== system WaveletTraj/Wavelet Trajectory/TrajGen4/Compute Join Coeffs/Derivative2 in tau1/Derivative ==
  Res : Inport  PortDimensions=1
  tau : Inport  Port=2  PortDimensions=1
  c : Inport  Port=3  PortDimensions=c_maxsz
  N : Inport  Port=4  PortDimensions=1
  For Iterator : ForIterator  ResetStates=reset  IterationSource=external  IndexMode=Zero-based  IterationVariableDataType=int8
  Lookup Table : Lookup  InputValues=tval_fi  Table=Dphival_fi  LookUpMeth=Interpolation-Use End Values  RndMeth=Nearest  SaturateOnIntegerOverflow=on
  Memory : Memory  InheritSampleTime=on
  Product : Product  OutDataTypeStr=fixdt(1,w,f)  RndMeth=Nearest  SaturateOnIntegerOverflow=on
  Product2 : Product  Inputs=3  OutDataTypeStr=fixdt(1,w,f)  RndMeth=Nearest  SaturateOnIntegerOverflow=on
  Selector : Selector  IndexMode=Zero-based  InputPortWidth=c_maxsz  IndexOptions=Index vector (port)  Indices=[1 3]  OutputSizes=1
  Sum : Sum  Inputs=|+-  OutDataTypeStr=fixdt(1,w,f)  RndMeth=Nearest  SaturateOnIntegerOverflow=on
  Sum1 : Sum  Inputs=|++  OutDataTypeStr=fixdt(1,w,f)  RndMeth=Nearest  SaturateOnIntegerOverflow=on
  Dout : Outport  PortDimensions=1  InitialOutput=0
  wires:
  tau/1 -> Product/2
  Res/1 -> Product/1, Product2/1
  Sum/1 -> Lookup Table/1
  Product/1 -> Sum/1
  N/1 -> For Iterator/1
  For Iterator/1 -> Sum/2, Selector/2
  c/1 -> Selector/1
  Memory/1 -> Sum1/2
  Sum1/1 -> Dout/1, Memory/1
  Lookup Table/1 -> Product2/2
  Selector/1 -> Product2/3
  Product2/1 -> Sum1/1

== system WaveletTraj/Wavelet Trajectory/TrajGen4/Compute Join Coeffs/Position2 in tau1/Position ==
  Res : Inport  PortDimensions=1
  tau : Inport  Port=2  PortDimensions=1
  c : Inport  Port=3  PortDimensions=c_maxsz
  N : Inport  Port=4  PortDimensions=1
  For Iterator : ForIterator  ResetStates=reset  IterationSource=external  IndexMode=Zero-based  IterationVariableDataType=int8
  Lookup Table : Lookup  InputValues=tval_fi  Table=phival_fi  LookUpMeth=Interpolation-Use End Values  RndMeth=Nearest  SaturateOnIntegerOverflow=on
  Memory : Memory  InheritSampleTime=on
  Product : Product  OutDataTypeStr=fixdt(1,w,f)  RndMeth=Nearest  SaturateOnIntegerOverflow=on
  Product1 : Product  OutDataTypeStr=fixdt(1,w,f)  RndMeth=Nearest  SaturateOnIntegerOverflow=on
  Selector : Selector  IndexMode=Zero-based  InputPortWidth=c_maxsz  IndexOptions=Index vector (port)  Indices=[1 3]  OutputSizes=1
  Sum : Sum  Inputs=|+-  OutDataTypeStr=fixdt(1,w,f)  RndMeth=Nearest  SaturateOnIntegerOverflow=on
  Sum1 : Sum  Inputs=|++  OutDataTypeStr=fixdt(1,w,f)  RndMeth=Nearest  SaturateOnIntegerOverflow=on
  out : Outport  PortDimensions=1  InitialOutput=0
  wires:
  Sum1/1 -> Memory/1, out/1
  Memory/1 -> Sum1/2
  Product1/1 -> Sum1/1
  Selector/1 -> Product1/2
  c/1 -> Selector/1
  Lookup Table/1 -> Product1/1
  For Iterator/1 -> Selector/2, Sum/2
  N/1 -> For Iterator/1
  Product/1 -> Sum/1
  Sum/1 -> Lookup Table/1
  Res/1 -> Product/1
  tau/1 -> Product/2

== system WaveletTraj/Wavelet Trajectory/TrajGen4/Compute Position/Position/Position ==
  Res : Inport  PortDimensions=1
  tau : Inport  Port=2  PortDimensions=1
  c : Inport  Port=3  PortDimensions=c_maxsz
  N : Inport  Port=4  PortDimensions=1
  For Iterator : ForIterator  ResetStates=reset  IterationSource=external  IndexMode=Zero-based  IterationVariableDataType=int8
  Lookup Table : Lookup  InputValues=tval_fi  Table=phival_fi  LookUpMeth=Interpolation-Use End Values  RndMeth=Nearest  SaturateOnIntegerOverflow=on
  Memory : Memory  InheritSampleTime=on
  Product : Product  OutDataTypeStr=fixdt(1,w,f)  RndMeth=Nearest  SaturateOnIntegerOverflow=on
  Product1 : Product  OutDataTypeStr=fixdt(1,w,f)  RndMeth=Nearest  SaturateOnIntegerOverflow=on
  Selector : Selector  IndexMode=Zero-based  InputPortWidth=c_maxsz  IndexOptions=Index vector (port)  Indices=[1 3]  OutputSizes=1
  Sum : Sum  Inputs=|+-  OutDataTypeStr=fixdt(1,w,f)  RndMeth=Nearest  SaturateOnIntegerOverflow=on
  Sum1 : Sum  Inputs=|++  OutDataTypeStr=fixdt(1,w,f)  RndMeth=Nearest  SaturateOnIntegerOverflow=on
  out : Outport  PortDimensions=1  InitialOutput=0
  wires:
  tau/1 -> Product/2
  Res/1 -> Product/1
  Sum/1 -> Lookup Table/1
  Product/1 -> Sum/1
  N/1 -> For Iterator/1
  For Iterator/1 -> Sum/2, Selector/2
  Lookup Table/1 -> Product1/1
  c/1 -> Selector/1
  Selector/1 -> Product1/2
  Product1/1 -> Sum1/1
  Memory/1 -> Sum1/2
  Sum1/1 -> out/1, Memory/1
